simulink model "control"  (R2023a)
settings: Solver=ode4  StartTime=0.0  StopTime=5  FixedStep=0.01  RelTol=1e-3
values from neighbouring files (symbols this model uses):
  A = [-6 -3 -2;22 5 10;-12 0 -7]    [eje4_par3.m]    (also in ejer1_par3.m = [9 -28 -40; 10 -28 -35;-4 11 12]; ejer2_par3.m = [8 -12 4;3 -4 1;-21 30 -11]; ejer3_par3.m = [101 -6 56;-121 4 -65;-208 12 -115]; ejer5_par3.m = [-16 -25 25; -7 -12 9;-17 -26 23])
  B = [-8;11;9]    [eje4_par3.m]    (also in ejer2_par3.m = [6;-6;-32]; ejer3_par3.m = [-1;2;2]; ejer5_par3.m = [-2;0;-2])
  x0 = [3;-9;8]    [eje4_par3.m]    (also in ejer2_par3.m = [-3,9,-10]; ejer3_par3.m = [-10;-7;-7])
settings Model: Creator=itzel  LastModifiedBy=userh
settings OptimizationCC: ReuseModelBlockBuffer=off

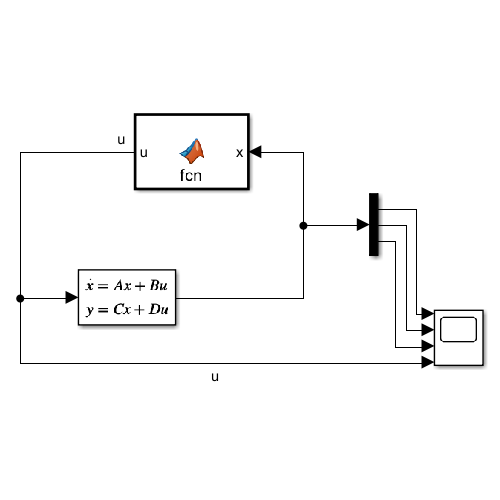
[thumbnail: Simulink's stored preview of the top-level diagram]
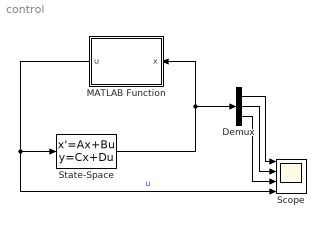
== system control ==
  Demux : Demux  Outputs=3
  MATLAB Function : MATLAB Function  TreatAsAtomicUnit=on
  Scope : Scope  NumInputPorts=4
  State-Space : StateSpace  A=A  B=B  C=eye(3)  D=zeros(3,1)  InitialCondition=x0
  wires:
  State-Space/1 -> MATLAB Function/1(x), Demux/1
  MATLAB Function/1(u) -> Scope/4, State-Space/1  "u"
  Demux/1 -> Scope/1
  Demux/3 -> Scope/3
  Demux/2 -> Scope/2

== matlab function control/MATLAB Function ==
  data: x input; u output
function u = fcn(x)
k1=-10.5;        
k2= 7;
k3=-3.5; 
rt=80;

u=-k1*x(1)-k2*x(2)-k3*x(3)+rt;
